simulink model "OfflineEstimator"  (R2020a)
settings: Solver=ode1be  StartTime=0.0  StopTime=simParams.duration.Value  FixedStep=0.00005  MaxStep=0.0005*sqrt(simParams.lengthScaleFactor.Value)  RelTol=1e-3  AbsTol=1e-3
undefined symbols (not defined in the file or in its folder): bridlePosVec, CMposVec, env, experimentalDataIsInput, externalDataIsInput, initPosKite, initVelKite, las, LEposIMU, linThrNodeCorrVec, NNodeTether, NNodeTether_cl, numObsThrNodes, obsLASphidotInit, obsLASphiInit, obsLASthetadotInit, obsLASthetaInit, ObsLink1DFlowVec, OBSTETHER, Obsthr, tow_start_time
libraries: vrlib x5, lineAngleSensor x5, dspsrcs4 x4, sharedutil x3, nodeDragForce_ul x3, nodeNetBuoyForce_ul x3, nodePosToLinkPos_ul x3, nodeSpringDamperForce_ul x3, eeGeneralControl x3, stateEstimation x3, dspsigops x3, thrNodeMass_ul x2
(part 2 of 2)

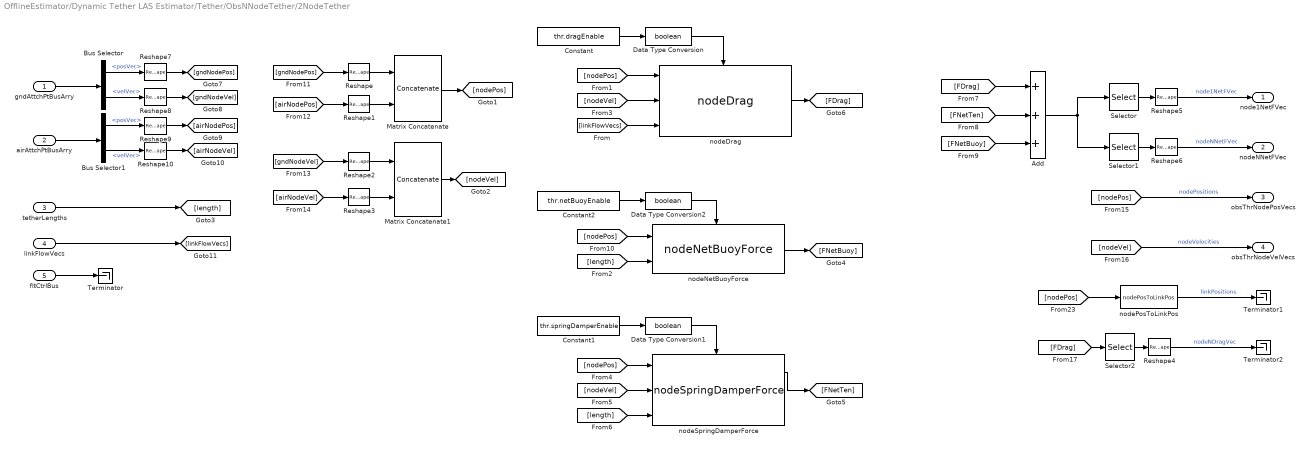
== system OfflineEstimator/Dynamic Tether LAS Estimator/Tether/ObsNNodeTether/2NodeTether ==
  gndAttchPtBusArry : Inport  OutDataTypeStr=Bus: thrAttachPtKinematicsBus
  airAttchPtBusArry : Inport  Port=2  OutDataTypeStr=Bus: thrAttachPtKinematicsBus
  tetherLengths : Inport  Port=3
  linkFlowVecs : Inport  Port=4
  fltCtrlBus : Inport  Port=5
  Add : Sum  Inputs=3
  Bus Selector : BusSelector  OutputSignals=posVec,velVec
  Bus Selector1 : BusSelector  OutputSignals=posVec,velVec
  Constant : Constant  Value=thr.dragEnable
  Constant1 : Constant  Value=thr.springDamperEnable
  Constant2 : Constant  Value=thr.netBuoyEnable
  Data Type Conversion : DataTypeConversion  OutDataTypeStr=boolean
  Data Type Conversion1 : DataTypeConversion  OutDataTypeStr=boolean
  Data Type Conversion2 : DataTypeConversion  OutDataTypeStr=boolean
  Matrix Concatenate : Concatenate  Mode=Multidimensional array  ConcatenateDimension=2
  Matrix Concatenate1 : Concatenate  Mode=Multidimensional array  ConcatenateDimension=2
  Reshape{,1..10} (11 alike) : Reshape  OutputDimensionality=Column vector (2-D)
  Selector : Selector  NumberOfDimensions=2  InputPortWidth=3  IndexOptions=Select all,Index vector (dialog)  Indices=[1 3],1  OutputSizes=1,1
  Selector1 : Selector  NumberOfDimensions=2  InputPortWidth=3  IndexOptions=Select all,Index vector (dialog)  Indices=[1 3],2  OutputSizes=1,1
  Selector2 : Selector  NumberOfDimensions=2  InputPortWidth=3  IndexOptions=Select all,Index vector (dialog)  Indices=[1 3],2  OutputSizes=1,1
  Terminator : Terminator
  Terminator1 : Terminator
  Terminator2 : Terminator
  nodeDrag : nodeDragForce_ul/nodeDrag  flowDensity=flowDensity  thrDiam=thr.diameter  dragCoeff=thr.dragCoeff
  nodeNetBuoyForce : nodeNetBuoyForce_ul/nodeNetBuoyForce  fluidDensity=flowDensity  tetherDensity=thr.density  diameter=thr.diameter  gravity=gravity
  nodePosToLinkPos : nodePosToLinkPos_ul/nodePosToLinkPos  SystemSampleTime=-1  Latency=0  AutoFrameSizeCalculation=off
  nodeSpringDamperForce : nodeSpringDamperForce_ul/nodeSpringDamperForce  mass=thr.vehicleMass  zeta=thr.dampingRatio  diameter=thr.diameter  youngsMod=thr.youngsMod
  node1NetFVec : Outport  VectorParamsAs1DForOutWhenUnconnected=off
  nodeNNetFVec : Outport  Port=2  VectorParamsAs1DForOutWhenUnconnected=off
  obsThrNodePosVecs : Outport  Port=3  VectorParamsAs1DForOutWhenUnconnected=off
  obsThrNodeVelVecs : Outport  Port=4  VectorParamsAs1DForOutWhenUnconnected=off
  wires:
  Matrix Concatenate/1 -> [nodePos]
  [nodePos] -> obsThrNodePosVecs/1  "nodePositions"
  [FNetBuoy] -> Add/3
  Reshape6/1 -> nodeNNetFVec/1  "nodeNNetFVec"
  Reshape10/1 -> [airNodeVel]
  [nodePos] -> nodeNetBuoyForce/1
  Data Type Conversion2/1 -> nodeNetBuoyForce/Enable
  Selector/1 -> Reshape5/1
  gndAttchPtBusArry/1 -> Bus Selector/1
  Bus Selector/2 -> Reshape8/1  "<velVec>"
  Reshape7/1 -> [gndNodePos]
  Selector2/1 -> Reshape4/1
  Reshape4/1 -> Terminator2/1  "nodeNDragVec"
  nodePosToLinkPos/1 -> Terminator1/1  "linkPositions"
  [FNetTen] -> Add/2
  [nodeVel] -> obsThrNodeVelVecs/1  "nodeVelocities"
  fltCtrlBus/1 -> Terminator/1
  Constant1/1 -> Data Type Conversion1/1
  tetherLengths/1 -> [length]
  Selector1/1 -> Reshape6/1
  Data Type Conversion1/1 -> nodeSpringDamperForce/Enable
  Reshape/1 -> Matrix Concatenate/1
  Reshape8/1 -> [gndNodeVel]
  [nodePos] -> nodeDrag/1
  Reshape9/1 -> [airNodePos]
  [nodeVel] -> nodeDrag/2
  Reshape5/1 -> node1NetFVec/1  "node1NetFVec"
  [length] -> nodeNetBuoyForce/2
  nodeSpringDamperForce/1 -> [FNetTen]
  nodeDrag/1 -> [FDrag]
  Add/1 -> Selector1/1, Selector/1
  [nodeVel] -> nodeSpringDamperForce/2
  nodeNetBuoyForce/1 -> [FNetBuoy]
  Bus Selector/1 -> Reshape7/1  "<posVec>"
  Data Type Conversion/1 -> nodeDrag/Enable
  [nodePos] -> nodePosToLinkPos/1
  Reshape1/1 -> Matrix Concatenate/2
  Bus Selector1/1 -> Reshape9/1  "<posVec>"
  [length] -> nodeSpringDamperForce/3
  Bus Selector1/2 -> Reshape10/1  "<velVec>"
  [airNodeVel] -> Reshape3/1
  Constant/1 -> Data Type Conversion/1
  Matrix Concatenate1/1 -> [nodeVel]
  [FDrag] -> Add/1
  [airNodePos] -> Reshape1/1
  [nodePos] -> nodeSpringDamperForce/1
  airAttchPtBusArry/1 -> Bus Selector1/1
  [gndNodeVel] -> Reshape2/1
  [gndNodePos] -> Reshape/1
  Constant2/1 -> Data Type Conversion2/1
  [FDrag] -> Selector2/1
  Reshape3/1 -> Matrix Concatenate1/2
  linkFlowVecs/1 -> [linkFlowVecs]
  Reshape2/1 -> Matrix Concatenate1/1
  [linkFlowVecs] -> nodeDrag/3

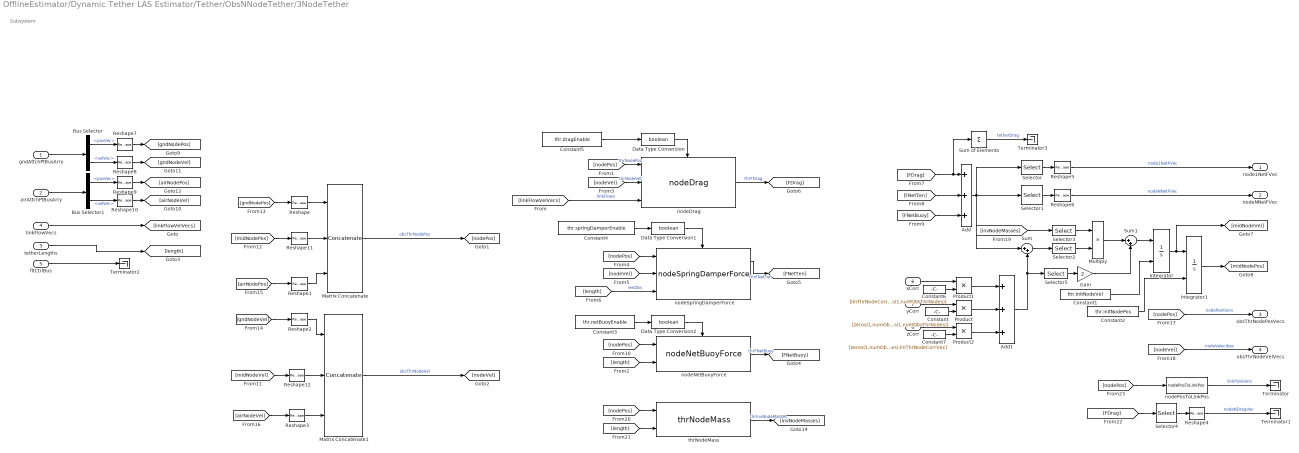
== system OfflineEstimator/Dynamic Tether LAS Estimator/Tether/ObsNNodeTether/3NodeTether ==
  note: Subsystem
  gndAttchPtBusArry : Inport  OutDataTypeStr=Bus: thrAttachPtKinematicsBus
  airAttchPtBusArry : Inport  Port=2  OutDataTypeStr=Bus: thrAttachPtKinematicsBus
  tetherLengths : Inport  Port=3
  linkFlowVecs : Inport  Port=4
  fltCtrlBus : Inport  Port=5
  xCorr : Inport  Port=6
  yCorr : Inport  Port=7
  zCorr : Inport  Port=8
  Add : Sum  Inputs=3
  Add1 : Sum  Inputs=3
  Bus Selector : BusSelector  OutputSignals=posVec,velVec
  Bus Selector1 : BusSelector  OutputSignals=posVec,velVec
  Constant : Constant  Value=[zeros(1,numObsThrNodes);linThrNodeCorrVec;zeros(1,numObsThrNodes)]
  Constant1 : Constant  Value=thr.initNodeVel
  Constant2 : Constant  Value=thr.initNodePos
  Constant3 : Constant  Value=thr.netBuoyEnable
  Constant4 : Constant  Value=thr.springDamperEnable
  Constant5 : Constant  Value=thr.dragEnable
  Constant6 : Constant  Value=[linThrNodeCorrVec;zeros(1,numObsThrNodes);zeros(1,numObsThrNodes)]
  Constant7 : Constant  Value=[zeros(1,numObsThrNodes);zeros(1,numObsThrNodes);linThrNodeCorrVec]
  Data Type Conversion : DataTypeConversion  OutDataTypeStr=boolean
  Data Type Conversion1 : DataTypeConversion  OutDataTypeStr=boolean
  Data Type Conversion2 : DataTypeConversion  OutDataTypeStr=boolean
  Gain : Gain  Gain=2
  Integrator : Integrator  InitialConditionSource=external
  Integrator1 : Integrator  InitialConditionSource=external
  Matrix Concatenate : Concatenate  NumInputs=3  Mode=Multidimensional array  ConcatenateDimension=2
  Matrix Concatenate1 : Concatenate  NumInputs=3  Mode=Multidimensional array  ConcatenateDimension=2
  Multiply : Product
  Product : Product
  Product1 : Product
  Product2 : Product
  Reshape{,1..12} (13 alike) : Reshape  OutputDimensionality=Column vector (2-D)
  Selector : Selector  NumberOfDimensions=2  InputPortWidth=3  IndexOptions=Select all,Index vector (dialog)  Indices=[1 3],1  OutputSizes=1,1
  Selector1 : Selector  NumberOfDimensions=2  InputPortWidth=3  IndexOptions=Select all,Starting index (dialog)  Indices=[1 3],numNodes  OutputSizes=1,1
  Selector2 : Selector  NumberOfDimensions=2  InputPortWidth=3  IndexOptions=Select all,Index vector (dialog)  Indices=[1 3],2:numNodes-1  OutputSizes=1,1
  Selector3 : Selector  NumberOfDimensions=2  InputPortWidth=3  IndexOptions=Select all,Index vector (dialog)  Indices=[1 3],2:numNodes-1  OutputSizes=1,1
  Selector4 : Selector  NumberOfDimensions=2  InputPortWidth=3  IndexOptions=Select all,Starting index (dialog)  Indices=[1 3],numNodes  OutputSizes=1,1
  Selector5 : Selector  NumberOfDimensions=2  InputPortWidth=3  IndexOptions=Select all,Index vector (dialog)  Indices=[1 3],2:numNodes-1  OutputSizes=1,1
  Sum : Sum  Inputs=|++
  Sum of Elements : Sum  Inputs=+  CollapseMode=Specified dimension  CollapseDim=2
  Sum1 : Sum  Inputs=|++
  Terminator{,1..3} (4 alike) : Terminator
  nodeDrag : nodeDragForce_ul/nodeDrag  flowDensity=flowDensity  thrDiam=thr.diameter  dragCoeff=thr.dragCoeff
  nodeNetBuoyForce : nodeNetBuoyForce_ul/nodeNetBuoyForce  fluidDensity=flowDensity  tetherDensity=thr.density  diameter=thr.diameter  gravity=gravity
  nodePosToLinkPos : nodePosToLinkPos_ul/nodePosToLinkPos  SystemSampleTime=-1  Latency=0  AutoFrameSizeCalculation=off
  nodeSpringDamperForce : nodeSpringDamperForce_ul/nodeSpringDamperForce  mass=thr.vehicleMass  zeta=thr.dampingRatio  diameter=thr.diameter  youngsMod=thr.youngsMod
  thrNodeMass : thrNodeMass_ul/thrNodeMass  tetherDensity=thr.density  diameter=thr.diameter
  node1NetFVec : Outport  VectorParamsAs1DForOutWhenUnconnected=off
  nodeNNetFVec : Outport  Port=2  VectorParamsAs1DForOutWhenUnconnected=off
  obsThrNodePosVecs : Outport  Port=3  VectorParamsAs1DForOutWhenUnconnected=off
  obsThrNodeVelVecs : Outport  Port=4  VectorParamsAs1DForOutWhenUnconnected=off
  wires:
  Reshape12/1 -> Matrix Concatenate1/2
  Reshape11/1 -> Matrix Concatenate/2
  Reshape4/1 -> Terminator1/1  "nodeNDragVec"
  [nodeVel] -> obsThrNodeVelVecs/1  "nodeVelocities"
  nodePosToLinkPos/1 -> Terminator/1  "linkPositions"
  [gndNodePos] -> Reshape/1
  Constant1/1 -> Integrator/2
  Integrator1/1 -> [midNodePos]
  [midNodePos] -> Reshape11/1
  Reshape9/1 -> [airNodePos]
  [nodePos] -> nodeSpringDamperForce/1
  Selector/1 -> Reshape5/1
  Reshape1/1 -> Matrix Concatenate/3
  [airNodeVel] -> Reshape3/1
  [nodeVel] -> nodeSpringDamperForce/2
  [nodePos] -> nodeDrag/1  "thrNodePos"
  [invNodeMasses] -> Selector3/1
  Reshape2/1 -> Matrix Concatenate1/1
  [FDrag] -> Add/1, Sum of Elements/1
  nodeSpringDamperForce/1 -> [FNetTen]  "thrFNetTen"
  [nodeVel] -> nodeDrag/2  "thrNodeVel"
  nodeNetBuoyForce/1 -> [FNetBuoy]  "thrFNetBuoy"
  Bus Selector/1 -> Reshape7/1  "<posVec>"
  Selector4/1 -> Reshape4/1
  tetherLengths/1 -> [length]
  [length] -> nodeSpringDamperForce/3  "lenObs"
  Bus Selector/2 -> Reshape8/1  "<velVec>"
  Multiply/1 -> Sum1/1
  Selector1/1 -> Reshape6/1
  Selector2/1 -> Multiply/2
  Bus Selector1/1 -> Reshape9/1  "<posVec>"
  [nodePos] -> nodeNetBuoyForce/1
  Reshape7/1 -> [gndNodePos]
  Integrator/1 -> [midNodeVel], Integrator1/1
  [airNodePos] -> Reshape1/1
  airAttchPtBusArry/1 -> Bus Selector1/1
  Reshape3/1 -> Matrix Concatenate1/3
  Bus Selector1/2 -> Reshape10/1  "<velVec>"
  Matrix Concatenate/1 -> [nodePos]  "obsThrNodePos"
  gndAttchPtBusArry/1 -> Bus Selector/1
  Reshape8/1 -> [gndNodeVel]
  [FNetTen] -> Add/2
  [FDrag] -> Selector4/1
  [nodePos] -> obsThrNodePosVecs/1  "nodePositions"
  [nodePos] -> thrNodeMass/1
  Sum of Elements/1 -> Terminator3/1  "tetherDrag"
  Add/1 -> Sum/1, Selector/1, Selector1/1
  Matrix Concatenate1/1 -> [nodeVel]  "obsThrNodeVel"
  fltCtrlBus/1 -> Terminator2/1
  [midNodeVel] -> Reshape12/1
  Data Type Conversion1/1 -> nodeSpringDamperForce/Enable
  Selector3/1 -> Multiply/1
  [length] -> nodeNetBuoyForce/2
  Reshape6/1 -> nodeNNetFVec/1  "nodeNNetFVec"
  thrNodeMass/1 -> [invNodeMasses]  "thrInvNodeMasses"
  Data Type Conversion/1 -> nodeDrag/Enable
  Data Type Conversion2/1 -> nodeNetBuoyForce/Enable
  linkFlowVecs/1 -> [linkFlowVelVecs]
  Constant2/1 -> Integrator1/2
  Constant5/1 -> Data Type Conversion/1
  [nodePos] -> nodePosToLinkPos/1
  Reshape10/1 -> [airNodeVel]
  Constant4/1 -> Data Type Conversion1/1
  Constant3/1 -> Data Type Conversion2/1
  [linkFlowVelVecs] -> nodeDrag/3  "linkFlows"
  [length] -> thrNodeMass/2
  [gndNodeVel] -> Reshape2/1
  nodeDrag/1 -> [FDrag]  "thrFDrag"
  Reshape/1 -> Matrix Concatenate/1
  [FNetBuoy] -> Add/3
  Reshape5/1 -> node1NetFVec/1  "node1NetFVec"
  yCorr/1 -> Product/1
  Constant/1 -> Product/2
  Product1/1 -> Add1/1
  Product/1 -> Add1/2
  Product2/1 -> Add1/3
  Constant7/1 -> Product2/2
  Constant6/1 -> Product1/2
  xCorr/1 -> Product1/1
  zCorr/1 -> Product2/1
  Sum/1 -> Selector2/1
  Gain/1 -> Sum1/2
  Selector5/1 -> Gain/1
  Add1/1 -> Sum/2, Selector5/1
  Sum1/1 -> Integrator/1

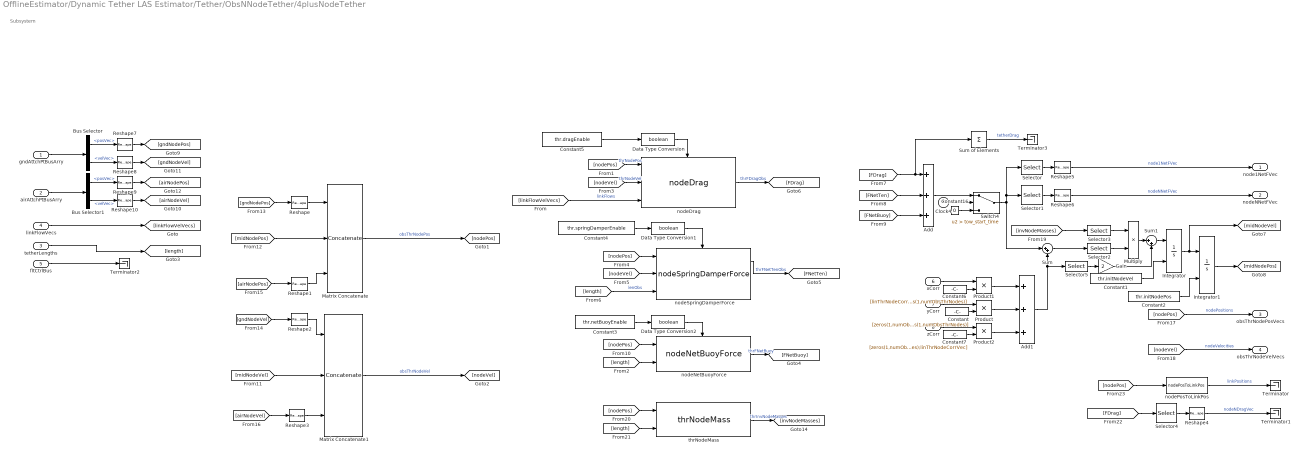
== system OfflineEstimator/Dynamic Tether LAS Estimator/Tether/ObsNNodeTether/4plusNodeTether ==
  note: Subsystem
  gndAttchPtBusArry : Inport  OutDataTypeStr=Bus: thrAttachPtKinematicsBus
  airAttchPtBusArry : Inport  Port=2  OutDataTypeStr=Bus: thrAttachPtKinematicsBus
  tetherLengths : Inport  Port=3
  linkFlowVecs : Inport  Port=4
  fltCtrlBus : Inport  Port=5
  xCorr : Inport  Port=6
  yCorr : Inport  Port=7
  zCorr : Inport  Port=8
  Add : Sum  Inputs=3
  Add1 : Sum  Inputs=3
  Bus Selector : BusSelector  OutputSignals=posVec,velVec
  Bus Selector1 : BusSelector  OutputSignals=posVec,velVec
  Clock4 : Clock
  Constant : Constant  Value=[zeros(1,numObsThrNodes);linThrNodeCorrVec;zeros(1,numObsThrNodes)]
  Constant1 : Constant  Value=thr.initNodeVel
  Constant16 : Constant  Value=0
  Constant2 : Constant  Value=thr.initNodePos
  Constant3 : Constant  Value=thr.netBuoyEnable
  Constant4 : Constant  Value=thr.springDamperEnable
  Constant5 : Constant  Value=thr.dragEnable
  Constant6 : Constant  Value=[linThrNodeCorrVec;zeros(1,numObsThrNodes);zeros(1,numObsThrNodes)]
  Constant7 : Constant  Value=[zeros(1,numObsThrNodes);zeros(1,numObsThrNodes);linThrNodeCorrVec]
  Data Type Conversion : DataTypeConversion  OutDataTypeStr=boolean
  Data Type Conversion1 : DataTypeConversion  OutDataTypeStr=boolean
  Data Type Conversion2 : DataTypeConversion  OutDataTypeStr=boolean
  Gain : Gain  Gain=2
  Integrator : Integrator  InitialConditionSource=external
  Integrator1 : Integrator  InitialConditionSource=external
  Matrix Concatenate : Concatenate  NumInputs=3  Mode=Multidimensional array  ConcatenateDimension=2
  Matrix Concatenate1 : Concatenate  NumInputs=3  Mode=Multidimensional array  ConcatenateDimension=2
  Multiply : Product
  Product : Product
  Product1 : Product
  Product2 : Product
  Reshape{,1..10} (11 alike) : Reshape  OutputDimensionality=Column vector (2-D)
  Selector : Selector  NumberOfDimensions=2  InputPortWidth=3  IndexOptions=Select all,Index vector (dialog)  Indices=[1 3],1  OutputSizes=1,1
  Selector1 : Selector  NumberOfDimensions=2  InputPortWidth=3  IndexOptions=Select all,Starting index (dialog)  Indices=[1 3],numNodes  OutputSizes=1,1
  Selector2 : Selector  NumberOfDimensions=2  InputPortWidth=3  IndexOptions=Select all,Index vector (dialog)  Indices=[1 3],2:numNodes-1  OutputSizes=1,1
  Selector3 : Selector  NumberOfDimensions=2  InputPortWidth=3  IndexOptions=Select all,Index vector (dialog)  Indices=[1 3],2:numNodes-1  OutputSizes=1,1
  Selector4 : Selector  NumberOfDimensions=2  InputPortWidth=3  IndexOptions=Select all,Starting index (dialog)  Indices=[1 3],numNodes  OutputSizes=1,1
  Selector5 : Selector  NumberOfDimensions=2  InputPortWidth=3  IndexOptions=Select all,Index vector (dialog)  Indices=[1 3],2:numNodes-1  OutputSizes=1,1
  Sum : Sum  Inputs=|++
  Sum of Elements : Sum  Inputs=+  CollapseMode=Specified dimension  CollapseDim=2
  Sum1 : Sum  Inputs=|++
  Switch4 : Switch  Criteria=u2 > Threshold  Threshold=tow_start_time
  Terminator{,1..3} (4 alike) : Terminator
  nodeDrag : nodeDragForce_ul/nodeDrag  flowDensity=flowDensity  thrDiam=thr.diameter  dragCoeff=thr.dragCoeff
  nodeNetBuoyForce : nodeNetBuoyForce_ul/nodeNetBuoyForce  fluidDensity=flowDensity  tetherDensity=thr.density  diameter=thr.diameter  gravity=gravity
  nodePosToLinkPos : nodePosToLinkPos_ul/nodePosToLinkPos  SystemSampleTime=-1  Latency=0  AutoFrameSizeCalculation=off
  nodeSpringDamperForce : nodeSpringDamperForce_ul/nodeSpringDamperForce  mass=thr.vehicleMass  zeta=thr.dampingRatio  diameter=thr.diameter  youngsMod=thr.youngsMod
  thrNodeMass : thrNodeMass_ul/thrNodeMass  tetherDensity=thr.density  diameter=thr.diameter
  node1NetFVec : Outport  VectorParamsAs1DForOutWhenUnconnected=off
  nodeNNetFVec : Outport  Port=2  VectorParamsAs1DForOutWhenUnconnected=off
  obsThrNodePosVecs : Outport  Port=3  VectorParamsAs1DForOutWhenUnconnected=off
  obsThrNodeVelVecs : Outport  Port=4  VectorParamsAs1DForOutWhenUnconnected=off
  wires:
  Constant16/1 -> Switch4/3
  Clock4/1 -> Switch4/2
  Add/1 -> Switch4/1
  Reshape5/1 -> node1NetFVec/1  "node1NetFVec"
  [FNetBuoy] -> Add/3
  Reshape/1 -> Matrix Concatenate/1
  nodeDrag/1 -> [FDrag]  "thrFDragObs"
  [gndNodeVel] -> Reshape2/1
  [length] -> thrNodeMass/2
  [linkFlowVelVecs] -> nodeDrag/3  "linkFlows"
  Constant3/1 -> Data Type Conversion2/1
  Constant4/1 -> Data Type Conversion1/1
  Reshape10/1 -> [airNodeVel]
  [nodePos] -> nodePosToLinkPos/1
  Constant5/1 -> Data Type Conversion/1
  Constant2/1 -> Integrator1/2
  linkFlowVecs/1 -> [linkFlowVelVecs]
  Data Type Conversion2/1 -> nodeNetBuoyForce/Enable
  Data Type Conversion/1 -> nodeDrag/Enable
  thrNodeMass/1 -> [invNodeMasses]  "thrInvNodeMasses"
  Reshape6/1 -> nodeNNetFVec/1  "nodeNNetFVec"
  [length] -> nodeNetBuoyForce/2
  Selector3/1 -> Multiply/1
  Data Type Conversion1/1 -> nodeSpringDamperForce/Enable
  [midNodeVel] -> Matrix Concatenate1/2
  fltCtrlBus/1 -> Terminator2/1
  Matrix Concatenate1/1 -> [nodeVel]  "obsThrNodeVel"
  Switch4/1 -> Sum/1, Selector1/1, Selector/1
  Sum of Elements/1 -> Terminator3/1  "tetherDrag"
  [nodePos] -> thrNodeMass/1
  [nodePos] -> obsThrNodePosVecs/1  "nodePositions"
  [FDrag] -> Selector4/1
  [FNetTen] -> Add/2
  Reshape8/1 -> [gndNodeVel]
  gndAttchPtBusArry/1 -> Bus Selector/1
  Matrix Concatenate/1 -> [nodePos]  "obsThrNodePos"
  Bus Selector1/2 -> Reshape10/1  "<velVec>"
  Reshape3/1 -> Matrix Concatenate1/3
  airAttchPtBusArry/1 -> Bus Selector1/1
  [airNodePos] -> Reshape1/1
  Integrator/1 -> Integrator1/1, [midNodeVel]
  Reshape7/1 -> [gndNodePos]
  [nodePos] -> nodeNetBuoyForce/1
  Bus Selector1/1 -> Reshape9/1  "<posVec>"
  Selector2/1 -> Multiply/2
  Selector1/1 -> Reshape6/1
  Multiply/1 -> Sum1/1
  Bus Selector/2 -> Reshape8/1  "<velVec>"
  [length] -> nodeSpringDamperForce/3  "lenObs"
  tetherLengths/1 -> [length]
  Selector4/1 -> Reshape4/1
  Bus Selector/1 -> Reshape7/1  "<posVec>"
  nodeNetBuoyForce/1 -> [FNetBuoy]  "thrFNetBuoy"
  [nodeVel] -> nodeDrag/2  "thrNodeVel"
  nodeSpringDamperForce/1 -> [FNetTen]  "thrFNetTenObs"
  [FDrag] -> Sum of Elements/1, Add/1
  Reshape2/1 -> Matrix Concatenate1/1
  [invNodeMasses] -> Selector3/1
  [nodePos] -> nodeDrag/1  "thrNodePos"
  [nodeVel] -> nodeSpringDamperForce/2
  [airNodeVel] -> Reshape3/1
  Reshape1/1 -> Matrix Concatenate/3
  Selector/1 -> Reshape5/1
  [nodePos] -> nodeSpringDamperForce/1
  Reshape9/1 -> [airNodePos]
  [midNodePos] -> Matrix Concatenate/2
  Integrator1/1 -> [midNodePos]
  Constant1/1 -> Integrator/2
  [gndNodePos] -> Reshape/1
  nodePosToLinkPos/1 -> Terminator/1  "linkPositions"
  [nodeVel] -> obsThrNodeVelVecs/1  "nodeVelocities"
  Reshape4/1 -> Terminator1/1  "nodeNDragVec"
  Constant/1 -> Product/2
  yCorr/1 -> Product/1
  Add1/1 -> Selector5/1, Sum/2
  xCorr/1 -> Product1/1
  Constant6/1 -> Product1/2
  zCorr/1 -> Product2/1
  Constant7/1 -> Product2/2
  Product2/1 -> Add1/3
  Product/1 -> Add1/2
  Product1/1 -> Add1/1
  Sum/1 -> Selector2/1
  Sum1/1 -> Integrator/1
  Selector5/1 -> Gain/1
  Gain/1 -> Sum1/2
